simulink model "exptwo_final"  (R2022b)
settings: Solver=VariableStepAuto  StartTime=0.0  StopTime=10  RelTol=1e-3
undefined symbols (not defined in the file): sigbuilder_block
libraries: spsSeriesRLCBranchLib x11, spsVoltageMeasurementLib x5, spsPVArrayLib x3, spsDiodeLib x2, spsIGBTLib x2, spsCurrentMeasurementLib x1, spspowerguiLib x1
settings Model: Creator=mohua  LastModifiedBy=mohua

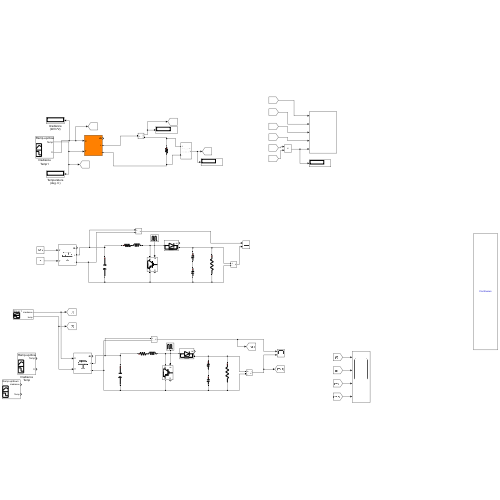
[thumbnail: Simulink's stored preview of the top-level diagram]
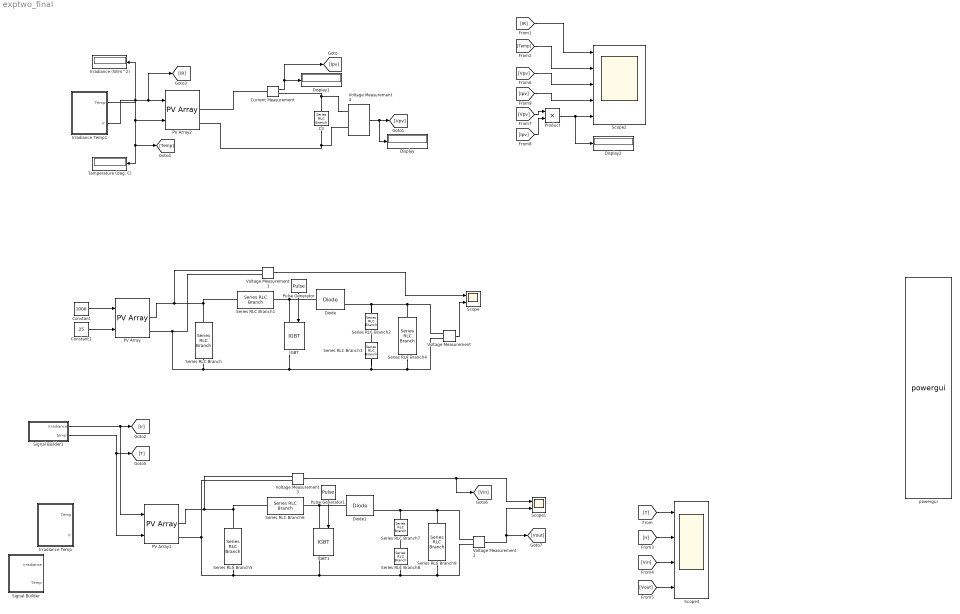
== system exptwo_final ==
  C3 : spsSeriesRLCBranchLib/Series RLC Branch  LConnTagsString=__new0  RConnTagsString=__new0  BranchType=R  Resistance=2  Inductance=1.0  SetiL0=off  InitialCurrent=0  Capacitance=100e-6  Setx0=off  InitialVoltage=0  Measurements=Branch voltage
  Constant : Constant  Value=1000
  Constant1 : Constant  Value=25
  Current Measurement : spsCurrentMeasurementLib/Current Measurement  PhasorSimulation=off  OutputType=Complex  PSBequivalent=0
  Diode : spsDiodeLib/Diode  Ron=0.001  Lon=0  Vf=0.8  IC=0  UseSnubber=0  Rs=500  Cs=250e-9  Measurements=on
  Diode1 : spsDiodeLib/Diode  Ron=0.001  Lon=0  Vf=0.8  IC=0  UseSnubber=0  Rs=500  Cs=250e-9  Measurements=on
  Display : Display
  Display1 : Display
  Display2 : Display
  IGBT : spsIGBTLib/IGBT  Ron=0.001  Lon=0  Vf=1  Tf=1e-6  Tt=2e-6  IC=0  Rs=1e5  Cs=inf  Measurements=on
  IGBT1 : spsIGBTLib/IGBT  Ron=0.001  Lon=0  Vf=1  Tf=1e-6  Tt=2e-6  IC=0  Rs=1e5  Cs=inf  Measurements=on
  Irradiance (W/m^2) : Display
      settings: Format=bank  Decimation=1000
  Irradiance Temp : Subsystem  Tag=STV Subsys  LoadFcn=sigbuilder_block('load');  StartFcn=sigbuilder_block('start');  StopFcn=sigbuilder_block('stop');  ClipboardFcn=sigbuilder_block('clipboard');  mask(Sigbuilder block){tuvar=[0:10]}
      mask help: Sigbuilder GUI
      mask init:
      | if ~strcmp(get_param(bdroot(gcbh),'SimulationStatus'),'stopped') tuvar = sigbuilder_block('maskInit'); end
      settings: CopyFcn=sigbuilder_block('copy');  DeleteFcn=sigbuilder_block('delete');  ModelCloseFcn=sigbuilder_block('modelClose');  PreSaveFcn=sigbuilder_block('preSave');  PauseFcn=sigbuilder_block('pause')  ContinueFcn=sigbuilder_block('continue')  NameChangeFcn=sigbuilder_block('namechange');  OpenFcn=sigbuilder_block('open',[5.4 36.6 1141.2 516.6 ]);  CloseFcn=sigbuilder_block('close');
      mask Display: plot(0, 0, 100, 100,[2, 2, 32, 32, 2], [68, 8, 8, 68, 68],[32, 2], [38, 38], [32, 19, 2],[53, 60, 44], [32, 17, 17, 2],[16, 16, 31, 31]);txt = getActiveGroup(gcbh);text(2, 100, txt,'verticalAlignment', 'top');
  Irradiance Temp1 : Subsystem  Tag=STV Subsys  LoadFcn=sigbuilder_block('load');  StartFcn=sigbuilder_block('start');  StopFcn=sigbuilder_block('stop');  ClipboardFcn=sigbuilder_block('clipboard');  mask(Sigbuilder block){tuvar=[0:10]}
      mask help: Sigbuilder GUI
      mask init:
      | if ~strcmp(get_param(bdroot(gcbh),'SimulationStatus'),'stopped') tuvar = sigbuilder_block('maskInit'); end
      settings: CopyFcn=sigbuilder_block('copy');  DeleteFcn=sigbuilder_block('delete');  ModelCloseFcn=sigbuilder_block('modelClose');  PreSaveFcn=sigbuilder_block('preSave');  PauseFcn=sigbuilder_block('pause')  ContinueFcn=sigbuilder_block('continue')  NameChangeFcn=sigbuilder_block('namechange');  OpenFcn=sigbuilder_block('open',[5.4 36.6 1141.2 516.6 ]);  CloseFcn=sigbuilder_block('close');
      mask Display: plot(0, 0, 100, 100,[2, 2, 32, 32, 2], [68, 8, 8, 68, 68],[32, 2], [38, 38], [32, 19, 2],[53, 60, 44], [32, 17, 17, 2],[16, 16, 31, 31]);txt = getActiveGroup(gcbh);text(2, 100, txt,'verticalAlignment', 'top');
  PV Array : spsPVArrayLib/PV Array  Npar=40  Nser=10  PlotType=array @ 1000 W/m2 & specified temperatures  S_vec="[ 1000  500  100 ]"  Temp_C_vec="[ 45 25  ]"  ModuleName=User-defined  PlotWhenSelected=off  Pm=213.15  Ncell=60  Voc=36.3  Isc=7.84  Vm=29  Im=7.35  beta_Voc_pc=-0.36099  alpha_Isc_pc=0.102  beta_Voc=-0.13104  alpha_Isc=0.0079968  IL=7.8654  I0=2.9273e-10  nI=0.98119  Rsh=313.0553  Rs=0.39381  RobustModel=off  RobustCellTemperature=313.3991  BAL=on  Tc=1e-6  Tfilter=5e-5
  PV Array1 : spsPVArrayLib/PV Array  Npar=40  Nser=10  PlotType=array @ 1000 W/m2 & specified temperatures  S_vec="[ 1000  500  100 ]"  Temp_C_vec="[ 45 25  ]"  ModuleName=User-defined  PlotWhenSelected=off  Pm=213.15  Ncell=60  Voc=36.3  Isc=7.84  Vm=29  Im=7.35  beta_Voc_pc=-0.36099  alpha_Isc_pc=0.102  beta_Voc=-0.13104  alpha_Isc=0.0079968  IL=7.8654  I0=2.9273e-10  nI=0.98119  Rsh=313.0553  Rs=0.39381  RobustModel=off  RobustCellTemperature=313.3991  BAL=on  Tc=1e-6  Tfilter=5e-5
  PV Array2 : spsPVArrayLib/PV Array  Npar=40  Nser=10  PlotType=array @ 1000 W/m2 & specified temperatures  S_vec="[ 1000  500  100 ]"  Temp_C_vec="[ 45 25  ]"  ModuleName=User-defined  PlotWhenSelected=off  Pm=213.15  Ncell=60  Voc=36.3  Isc=7.84  Vm=29  Im=7.35  beta_Voc_pc=-0.36099  alpha_Isc_pc=0.102  beta_Voc=-0.13104  alpha_Isc=0.0079968  IL=7.8654  I0=2.9273e-10  nI=0.98119  Rsh=313.0553  Rs=0.39381  RobustModel=off  RobustCellTemperature=313.3991  BAL=off  Tc=1e-6  Tfilter=5e-5
  Product : Product
  Pulse Generator : DiscretePulseGenerator  PulseType=Time based  Period=1/10000  PulseWidth=30
  Pulse Generator1 : DiscretePulseGenerator  PulseType=Time based  Period=1/10000  PulseWidth=30
  Scope : Scope  NumInputPorts=2
  Scope1 : Scope  NumInputPorts=2
  Scope2 : Scope  NumInputPorts=5
  Scope3 : Scope  NumInputPorts=4
  Series RLC Branch : spsSeriesRLCBranchLib/Series RLC Branch  LConnTagsString=__new0  RConnTagsString=__new0  BranchType=C  Resistance=1  Inductance=1e-3  SetiL0=off  InitialCurrent=0  Capacitance=100e-6  Setx0=off  InitialVoltage=0  Measurements=None
  Series RLC Branch1 : spsSeriesRLCBranchLib/Series RLC Branch  LConnTagsString=__new0  RConnTagsString=__new0  BranchType=RL  Resistance=0.000001  Inductance=5e-3  SetiL0=off  InitialCurrent=0  Capacitance=100e-6  Setx0=off  InitialVoltage=0  Measurements=None
  Series RLC Branch{2..3,7..8} (4 alike) : spsSeriesRLCBranchLib/Series RLC Branch  LConnTagsString=__new0  RConnTagsString=__new0  BranchType=C  Resistance=1  Inductance=1e-3  SetiL0=off  InitialCurrent=0  Capacitance=100e-3  Setx0=off  InitialVoltage=0  Measurements=None
  Series RLC Branch4 : spsSeriesRLCBranchLib/Series RLC Branch  LConnTagsString=__new0  RConnTagsString=__new0  BranchType=R  Resistance=50  Inductance=1e-3  SetiL0=off  InitialCurrent=0  Capacitance=100e-6  Setx0=off  InitialVoltage=0  Measurements=None
  Series RLC Branch5 : spsSeriesRLCBranchLib/Series RLC Branch  LConnTagsString=__new0  RConnTagsString=__new0  BranchType=C  Resistance=1  Inductance=1e-3  SetiL0=off  InitialCurrent=0  Capacitance=100e-6  Setx0=off  InitialVoltage=0  Measurements=None
  Series RLC Branch6 : spsSeriesRLCBranchLib/Series RLC Branch  LConnTagsString=__new0  RConnTagsString=__new0  BranchType=RL  Resistance=0.000001  Inductance=5e-3  SetiL0=off  InitialCurrent=0  Capacitance=100e-6  Setx0=off  InitialVoltage=0  Measurements=None
  Series RLC Branch9 : spsSeriesRLCBranchLib/Series RLC Branch  LConnTagsString=__new0  RConnTagsString=__new0  BranchType=R  Resistance=50  Inductance=1e-3  SetiL0=off  InitialCurrent=0  Capacitance=100e-6  Setx0=off  InitialVoltage=0  Measurements=None
  Signal Builder : Subsystem  Tag=STV Subsys  LoadFcn=sigbuilder_block('load');  StartFcn=sigbuilder_block('start');  StopFcn=sigbuilder_block('stop');  ClipboardFcn=sigbuilder_block('clipboard');  mask(Sigbuilder block){tuvar=[0:10]}
      mask help: Simulink:masks:SigbuilderBlock_MD
      mask init:
      | if ~strcmp(get_param(bdroot(gcbh),'SimulationStatus'),'stopped') tuvar = sigbuilder_block('maskInit'); end
      settings: CopyFcn=sigbuilder_block('copy');  DeleteFcn=sigbuilder_block('delete');  ModelCloseFcn=sigbuilder_block('modelClose');  PreSaveFcn=sigbuilder_block('preSave');  PauseFcn=sigbuilder_block('pause');  ContinueFcn=sigbuilder_block('continue');  NameChangeFcn=sigbuilder_block('namechange');  OpenFcn=sigbuilder_block('open',[132 139.2 550.8 400.2 ]);  CloseFcn=sigbuilder_block('close');
      mask Display: plot(0, 0, 100, 100,[2, 2, 32, 32, 2], [68, 8, 8, 68, 68],[32, 2], [38, 38], [32, 19, 2],[53, 60, 44], [32, 17, 17, 2],[16, 16, 31, 31]);txt = getActiveGroup(gcbh);text(2, 100, txt,'verticalAlignment', 'top');
  Signal Builder1 : Subsystem  Tag=STV Subsys  LoadFcn=sigbuilder_block('load');  StartFcn=sigbuilder_block('start');  StopFcn=sigbuilder_block('stop');  ClipboardFcn=sigbuilder_block('clipboard');  mask(Sigbuilder block){tuvar=[0:10]}
      mask help: Simulink:masks:SigbuilderBlock_MD
      mask init:
      | if ~strcmp(get_param(bdroot(gcbh),'SimulationStatus'),'stopped') tuvar = sigbuilder_block('maskInit'); end
      settings: CopyFcn=sigbuilder_block('copy');  DeleteFcn=sigbuilder_block('delete');  ModelCloseFcn=sigbuilder_block('modelClose');  PreSaveFcn=sigbuilder_block('preSave');  PauseFcn=sigbuilder_block('pause');  ContinueFcn=sigbuilder_block('continue');  NameChangeFcn=sigbuilder_block('namechange');  OpenFcn=sigbuilder_block('open',[437.6 199.2 550.4 400 ]);  CloseFcn=sigbuilder_block('close');
      mask Display: plot(0, 0, 100, 100,[2, 2, 32, 32, 2], [68, 8, 8, 68, 68],[32, 2], [38, 38], [32, 19, 2],[53, 60, 44], [32, 17, 17, 2],[16, 16, 31, 31]);txt = getActiveGroup(gcbh);text(2, 100, txt,'verticalAlignment', 'top');
  Temperature (deg. C) : Display
      settings: Format=bank  Decimation=1000
  Voltage Measurement{,1..4} (5 alike) : spsVoltageMeasurementLib/Voltage Measurement  PhasorSimulation=off  OutputType=Complex  PSBequivalent=0
  powergui : spspowerguiLib/powergui  Priority=1  SimulationMode=Continuous  SampleTime=50e-6  frequency=60  Iterations=50  frequencyindice=0  Pbase=100e6  ErrMax=1e-4  UnitsV=kV  UnitsW=MW  buscounter=0  FunctionMessages=off  echomessages=off  EnableUseOfTLC=off  CurrentSourceSwitches=off  DisableSnubberDevices=off  DisableRonSwitches=off  DisableVfSwitches=off  DisplayEquations=off  AutomaticDiscreteSolvers=off  SolverType=Tustin/Backward Euler (TBE)  Interpol=off  ExternalGateDelay=off  methode=off  Ts=100  x0status=blocks  SPID=on  SwTol=0  HookPort=off  NonlinearTolerance=1e-4  nMaxIteration=100  ContinueOnMaxIteration=off  RestoreLinks=warning  ResistiveCurrentMeasurement=off  Frange=[0:2:500]  Ylog=off  Xlog=on  ShowGrid=off  save=off  variable=ZData  structure=0  ZoomFFT=off  StartTime=0.0  cycles=1  DisplayStyle=1  fundamental=60  FreqAxis=off  MaxFrequency=1000  frequencyindicesteady=1  RmsSteady=1  display=off
  wires:
  Voltage Measurement1/1 -> Scope/1
  Voltage Measurement/1 -> Scope/2
  Constant/1 -> PV Array/1
  Constant1/1 -> PV Array/2
  Pulse Generator/1 -> IGBT/1
  Pulse Generator1/1 -> IGBT1/1
  Voltage Measurement2/1 -> Scope1/2, [Vout]
  Voltage Measurement3/1 -> [Vin], Scope1/1
  [Vpv] -> Scope2/3
  [Vpv] -> Product/1
  Product/1 -> Display2/1, Scope2/5
  [Ipv] -> Product/2
  Irradiance Temp1/2(Ir) -> PV Array2/1, [IR], Irradiance (W/m^2)/1
  [Ipv] -> Scope2/4
  Current Measurement/1 -> Display1/1, [Ipv]
  [IR] -> Scope2/1
  [Temp] -> Scope2/2
  Voltage Measurement4/1 -> Display/1, [Vpv]
  Irradiance Temp1/1(Temp) -> PV Array2/2, [Temp], Temperature (deg. C)/1
  [T] -> Scope3/1
  [Ir] -> Scope3/2
  [Vin] -> Scope3/3
  [Vout] -> Scope3/4
  Signal Builder1/1(irradiance) -> [Ir], PV Array1/1
  Signal Builder1/2(temp) -> PV Array1/2, [T]
  connections:
  Series RLC Branch/LConn1 -- Series RLC Branch1/LConn1 -- Voltage Measurement1/LConn1 -- PV Array/RConn1
  Series RLC Branch/RConn1 -- Series RLC Branch4/RConn1 -- Voltage Measurement/LConn2 -- Series RLC Branch3/RConn1 -- IGBT/RConn1 -- Voltage Measurement1/LConn2 -- PV Array/RConn2
  IGBT/LConn1 -- Diode/LConn1 -- Series RLC Branch1/RConn1
  Series RLC Branch2/LConn1 -- Series RLC Branch4/LConn1 -- Voltage Measurement/LConn1 -- Diode/RConn1
  Series RLC Branch3/LConn1 -- Series RLC Branch2/RConn1
  Series RLC Branch5/LConn1 -- PV Array1/RConn1 -- Voltage Measurement3/LConn1 -- Series RLC Branch6/LConn1
  Series RLC Branch9/RConn1 -- Voltage Measurement2/LConn2 -- Voltage Measurement3/LConn2 -- PV Array1/RConn2 -- Series RLC Branch5/RConn1 -- IGBT1/RConn1 -- Series RLC Branch8/RConn1
  Diode1/LConn1 -- Series RLC Branch6/RConn1 -- IGBT1/LConn1
  Series RLC Branch9/LConn1 -- Voltage Measurement2/LConn1 -- Diode1/RConn1 -- Series RLC Branch7/LConn1
  Series RLC Branch8/LConn1 -- Series RLC Branch7/RConn1
  Voltage Measurement4/LConn2 -- C3/RConn1 -- PV Array2/RConn2
  Voltage Measurement4/LConn1 -- C3/LConn1 -- Current Measurement/RConn1
  Current Measurement/LConn1 -- PV Array2/RConn1

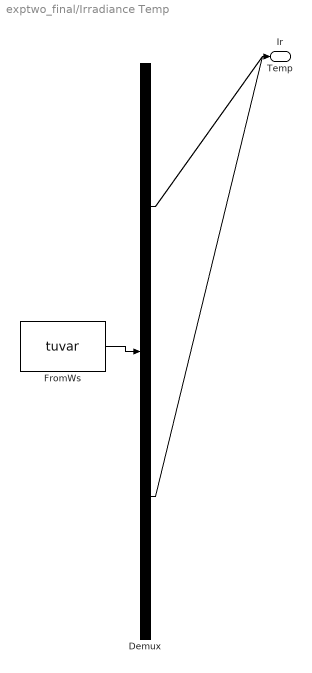
== system exptwo_final/Irradiance Temp ==
  Demux : Demux  Tag=STV Demux  Outputs=2
      settings: DisplayOption=none
  FromWs : FromWorkspace  Tag=STV FromWs  VariableName=tuvar
      SigBuilderData=|
      | common.afterFinalStr = 'Extrapolate'
      | common.sampleTime = '0'
      | dataSet(1).timeRange = [0 2]
      | dataSet(1).name = 'Constant Irradiance'
      | dataSet(2).timeRange = [0 2]
      | dataSet(2).name = 'Step Irradiance'
      | dataSet(3).timeRange = [0 3]
      | dataSet(3).name = 'Ramp-up/down Irradiance'
      | sbobj.Groups(1).Name = 'Constant Irradiance'
      | sbobj.Groups(1).Signals(1).Name = 'Temp'
      | sbobj.Groups(1).Signals(1).XData = [0 1 1 2]
      | sbobj.Groups(1).Signals(1).YData = [0 0 1 1]
      | sbobj.Groups(1).Signals(2).Name = 'Ir'
      | sbobj.Groups(1).Signals(2).XData = [0 2]
      | sbobj.Groups(1).Signals(2).YData = [1000 1000]
      | sbobj.Groups(1).TimeRange = [0 2]
      | sbobj.Groups(2).Name = 'Step Irradiance'
      | sbobj.Groups(2).Signals(1).Name = 'Temp'
      | sbobj.Groups(2).Signals(1).XData = [0 1 1 2]
      | sbobj.Groups(2).Signals(1).YData = [0 0 1 1]
      | sbobj.Groups(2).Signals(2).Name = 'Ir'
      | sbobj.Groups(2).Signals(2).XData = [0 0.252 0.252 2]
      | sbobj.Groups(2).Signals(2).YData = [600 600 1000 1000]
      | sbobj.Groups(2).TimeRange = [0 2]
      | sbobj.Groups(3).Name = 'Ramp-up/down Irradiance'
      | sbobj.Groups(3).Signals(1).Name = 'Temp'
      | sbobj.Groups(3).Signals(1).XData = [0 2 2 2.1 3]
      | sbobj.Groups(3).Signals(1).YData = [24.8 39 43.6 44.2 25.2]
      | sbobj.Groups(3).Signals(2).Name = 'Ir'
      | sbobj.Groups(3).Signals(2).XData = [0 0.6 1.1 1.2 1.7 1.7 3]
      | sbobj.Groups(3).Signals(2).YData = [1000 920 1040 1160 1085 1130 1040]
      | sbobj.Groups(3).TimeRange = [0 3]
  Temp : Outport  Tag=STV Outport  VectorParamsAs1DForOutWhenUnconnected=off
  Ir : Outport  Tag=STV Outport  Port=2  VectorParamsAs1DForOutWhenUnconnected=off
  wires:
  FromWs/1 -> Demux/1
  Demux/1 -> Temp/1
  Demux/2 -> Ir/1

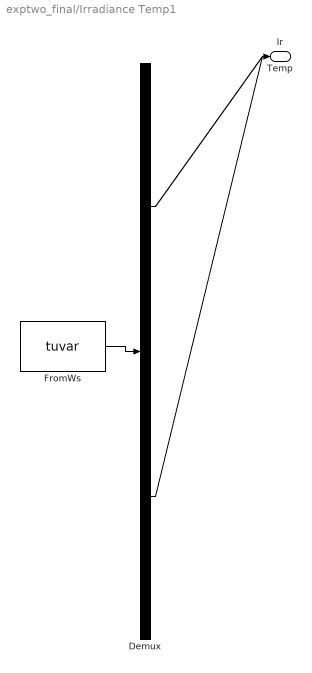
== system exptwo_final/Irradiance Temp1 ==
  Demux : Demux  Tag=STV Demux  Outputs=2
      settings: DisplayOption=none
  FromWs : FromWorkspace  Tag=STV FromWs  VariableName=tuvar
      SigBuilderData=|
      | common.afterFinalStr = 'Extrapolate'
      | common.sampleTime = '0'
      | dataSet(1).timeRange = [0 2]
      | dataSet(1).name = 'Constant Irradiance'
      | dataSet(2).timeRange = [0 2]
      | dataSet(2).name = 'Step Irradiance'
      | dataSet(3).timeRange = [0 3]
      | dataSet(3).name = 'Ramp-up/down Irradiance'
      | sbobj.Groups(1).Name = 'Constant Irradiance'
      | sbobj.Groups(1).Signals(1).Name = 'Temp'
      | sbobj.Groups(1).Signals(1).XData = [0 1 1 2]
      | sbobj.Groups(1).Signals(1).YData = [0 0 1 1]
      | sbobj.Groups(1).Signals(2).Name = 'Ir'
      | sbobj.Groups(1).Signals(2).XData = [0 2]
      | sbobj.Groups(1).Signals(2).YData = [1000 1000]
      | sbobj.Groups(1).TimeRange = [0 2]
      | sbobj.Groups(2).Name = 'Step Irradiance'
      | sbobj.Groups(2).Signals(1).Name = 'Temp'
      | sbobj.Groups(2).Signals(1).XData = [0 1 1 2]
      | sbobj.Groups(2).Signals(1).YData = [0 0 1 1]
      | sbobj.Groups(2).Signals(2).Name = 'Ir'
      | sbobj.Groups(2).Signals(2).XData = [0 0.252 0.252 2]
      | sbobj.Groups(2).Signals(2).YData = [600 600 1000 1000]
      | sbobj.Groups(2).TimeRange = [0 2]
      | sbobj.Groups(3).Name = 'Ramp-up/down Irradiance'
      | sbobj.Groups(3).Signals(1).Name = 'Temp'
      | sbobj.Groups(3).Signals(1).XData = [0 2 2 2.1 3]
      | sbobj.Groups(3).Signals(1).YData = [24.8 36.2 36.4 31.2 25.2]
      | sbobj.Groups(3).Signals(2).Name = 'Ir'
      | sbobj.Groups(3).Signals(2).XData = [0 0.6 1.1 1.2 1.7 3]
      | sbobj.Groups(3).Signals(2).YData = [1000 820 1010 850 1085 1000]
      | sbobj.Groups(3).TimeRange = [0 3]
  Temp : Outport  Tag=STV Outport  VectorParamsAs1DForOutWhenUnconnected=off
  Ir : Outport  Tag=STV Outport  Port=2  VectorParamsAs1DForOutWhenUnconnected=off
  wires:
  FromWs/1 -> Demux/1
  Demux/1 -> Temp/1
  Demux/2 -> Ir/1

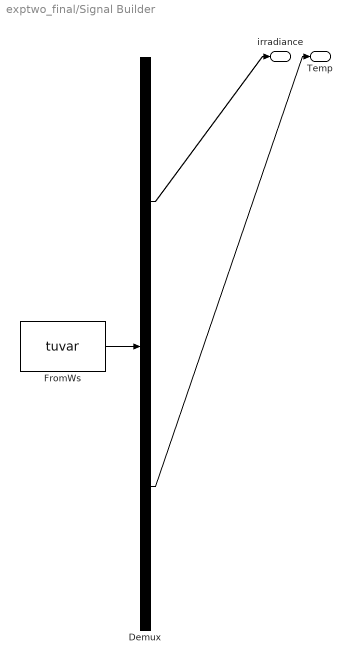
== system exptwo_final/Signal Builder ==
  Demux : Demux  Tag=STV Demux  Outputs=2
      settings: DisplayOption=none
  FromWs : FromWorkspace  Tag=STV FromWs  VariableName=tuvar
      SigBuilderData=|
      | common.afterFinalStr = 'Extrapolate'
      | common.sampleTime = 0
      | dataSet.timeRange = [0 10]
      | dataSet.name = 'Ramp up/down'
      | sbobj.Groups.Name = 'Ramp up/down'
      | sbobj.Groups.Signals(1).Name = 'irradiance'
      | sbobj.Groups.Signals(1).XData = [0 1 1 2 2 2.98 2.98 3.56 5 6 6.94 9.04 10]
      | sbobj.Groups.Signals(1).YData = [0.93 0.93 0.925 0.815 0.93 0.91 0.795 0.935 0.875 0.915 0.955 0.87 0.8]
      | sbobj.Groups.Signals(2).Name = 'Temp'
      | sbobj.Groups.Signals(2).XData = [0 1 2 3 4 5 5.95 6.95 7.95 9 10]
      | sbobj.Groups.Signals(2).YData = [0.21 0.4 0.79 0.79 0.44 0.7 0.33 0.53 0.71 0.71 0.21]
  irradiance : Outport  Tag=STV Outport
  Temp : Outport  Tag=STV Outport  Port=2
  wires:
  FromWs/1 -> Demux/1
  Demux/1 -> irradiance/1
  Demux/2 -> Temp/1

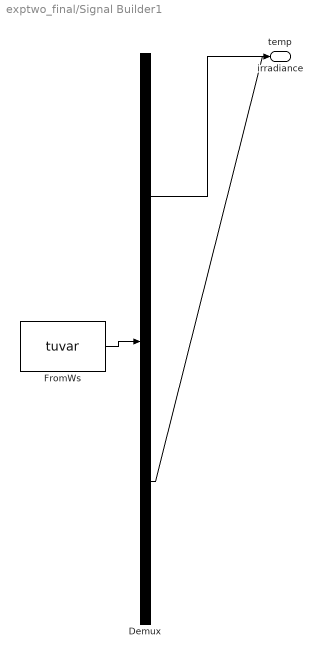
== system exptwo_final/Signal Builder1 ==
  Demux : Demux  Tag=STV Demux  Outputs=2
      settings: DisplayOption=none
  FromWs : FromWorkspace  Tag=STV FromWs  VariableName=tuvar
      SigBuilderData=|
      | common.afterFinalStr = 'Extrapolate'
      | common.sampleTime = 0
      | dataSet.timeRange = [0 10]
      | dataSet.name = 'Group 1'
      | sbobj.Groups.Name = 'Group 1'
      | sbobj.Groups.Signals(1).Name = 'irradiance'
      | sbobj.Groups.Signals(1).XData = [0 2.76 5 7.98 10]
      | sbobj.Groups.Signals(1).YData = [1000 1010 870 1260 1020]
      | sbobj.Groups.Signals(2).Name = 'temp'
      | sbobj.Groups.Signals(2).XData = [0 1.92 2.94 4.18 5.04 7.04 10]
      | sbobj.Groups.Signals(2).YData = [20 37 90 70 35 23 23]
  irradiance : Outport  Tag=STV Outport
  temp : Outport  Tag=STV Outport  Port=2
  wires:
  FromWs/1 -> Demux/1
  Demux/1 -> irradiance/1
  Demux/2 -> temp/1
